simulink model "hab"  (R2024b)
settings: Solver=VariableStepAuto  StartTime=0.0  StopTime=10  RelTol=1e-3
values from neighbouring files (symbols this model uses):
  g = 9.81    [constants.m]
  h = 20000    [constants.m]
  m_balloon = 500    [constants.m]
  m_gas = 1600    [constants.m]
  M_gas = 4.002602    [constants.m]
  m_payload = 1500    [constants.m]
  R = 8.314    [constants.m]
  up = [0 0 1]    [constants.m]
libraries: shared6dof x1, aerolibatmos2 x1
settings Model: Creator=Eduard Anton  LastModifiedBy=Eduard Anton

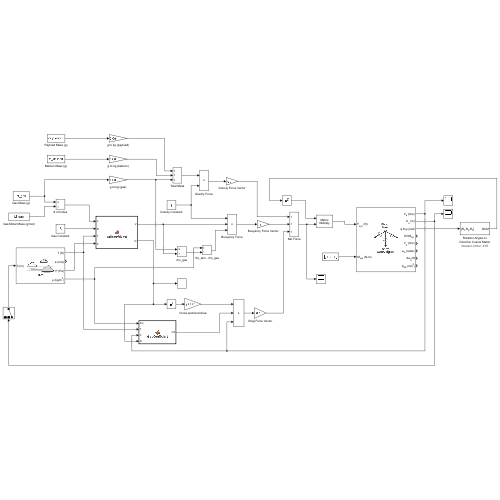
[thumbnail: Simulink's stored preview of the top-level diagram]
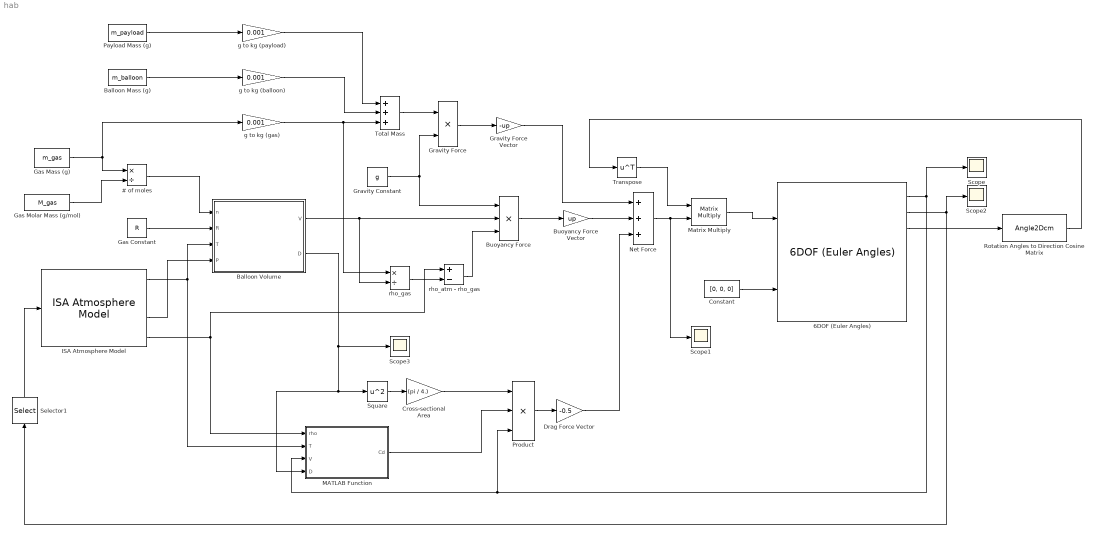
== system hab ==
  # of moles : Product  Inputs=*/
  6DOF (Euler Angles) : shared6dof/6DOF (Euler Angles)  units=Metric (MKS)  mtype=Fixed  rep=Euler Angles  xme_0=[0 0 h]  Vm_0=[0 0 0]  eul_0=[0 0 0]  pm_0=[0 0 0]  mass_0=1.0  mass_e=0.5  mass_f=2.0  inertia=eye(3)  inertia_e=eye(3)  inertia_f=2*eye(3)  k_quat=1.0  vre_flag=on  abi_flag=off  aMode=0  xme_statename=''  Vm_statename=''  eul_statename=''  quat_statename=''  pm_statename=''  mass_statename=''
  Balloon Mass (g) : Constant  Value=m_balloon
  Balloon Volume : MATLAB Function  TreatAsAtomicUnit=on
  Buoyancy Force : Product  Inputs=3
  Buoyancy Force Vector : Gain  Gain=up
  Constant : Constant  Value=[0, 0, 0]
  Cross-sectional Area : Gain  Gain=(pi / 4.)
  Drag Force Vector : Gain  Gain=-0.5
  Gas Constant : Constant  Value=R  VectorParams1D=off
  Gas Mass (g) : Constant  Value=m_gas
  Gas Molar Mass (g/mol) : Constant  Value=M_gas
  Gravity Constant : Constant  Value=g
  Gravity Force : Product
  Gravity Force Vector : Gain  Gain=-up
  ISA Atmosphere Model : aerolibatmos2/ISA Atmosphere Model  useExtended=on  action=Warning  custom=off  viscosityOut=off  g=9.80665  gamma=1.4  R=287.0531  L=0.0065  h_trop=11000  h_strat=20000  rho0=1.225  P0=101325  T0=288.15  h0=0  S=110.4  Tref=273.15  muref=1.716e-5
  MATLAB Function : MATLAB Function  TreatAsAtomicUnit=on
  Matrix Multiply : Product  Multiplication=Matrix(*)
  Net Force : Sum  Inputs=+++
  Payload Mass (g) : Constant  Value=m_payload
  Product : Product  Inputs=3
  Rotation Angles to Direction Cosine Matrix : Angle2Dcm  rotationOrder=XYZ
      settings: AttributesFormatString=Rotation Order: %<rotationOrder>
  Scope{,1..3} (4 alike) : Scope
  Selector1 : Selector  InputPortWidth=3  IndexOptions=Index vector (dialog)  Indices=3  OutputSizes=1
  Square : Math  Operator=square
  Total Mass : Sum  Inputs=+++
  Transpose : Math  Operator=transpose
  g to kg (balloon) : Gain  Gain=0.001
  g to kg (gas) : Gain  Gain=0.001
  g to kg (payload) : Gain  Gain=0.001
  rho_atm - rho_gas : Sum  Inputs=+-
  rho_gas : Product  Inputs=*/
  wires:
  ISA Atmosphere Model/1 -> Balloon Volume/3(T), MATLAB Function/2(T)
  ISA Atmosphere Model/3 -> Balloon Volume/4(P)
  Gas Constant/1 -> Balloon Volume/2(R)
  # of moles/1 -> Balloon Volume/1(n)
  ISA Atmosphere Model/4 -> rho_atm - rho_gas/1, MATLAB Function/1(rho)
  Gravity Constant/1 -> Buoyancy Force/1, Gravity Force/2
  Gas Mass (g)/1 -> g to kg (gas)/1, # of moles/1
  Gas Molar Mass (g/mol)/1 -> # of moles/2
  Balloon Volume/2(D) -> Scope3/1, MATLAB Function/4(D), Square/1
  Square/1 -> Cross-sectional Area/1
  Cross-sectional Area/1 -> Product/1
  MATLAB Function/1(Cd) -> Product/2
  Product/1 -> Drag Force Vector/1
  Constant/1 -> 6DOF (Euler Angles)/2
  g to kg (gas)/1 -> rho_gas/1, Total Mass/3
  Gravity Force/1 -> Gravity Force Vector/1
  Buoyancy Force/1 -> Buoyancy Force Vector/1
  6DOF (Euler Angles)/1 -> Product/3, MATLAB Function/3(V), Scope/1
  6DOF (Euler Angles)/2 -> Scope2/1, Selector1/1
  Balloon Volume/1(V) -> rho_gas/2, Buoyancy Force/2
  rho_gas/1 -> rho_atm - rho_gas/2
  rho_atm - rho_gas/1 -> Buoyancy Force/3
  Gravity Force Vector/1 -> Net Force/1
  Buoyancy Force Vector/1 -> Net Force/2
  Total Mass/1 -> Gravity Force/1
  Balloon Mass (g)/1 -> g to kg (balloon)/1
  g to kg (balloon)/1 -> Total Mass/2
  Payload Mass (g)/1 -> g to kg (payload)/1
  g to kg (payload)/1 -> Total Mass/1
  6DOF (Euler Angles)/3 -> Rotation Angles to Direction Cosine Matrix/1
  Net Force/1 -> Scope1/1, Matrix Multiply/2
  Rotation Angles to Direction Cosine Matrix/1 -> Transpose/1
  Transpose/1 -> Matrix Multiply/1
  Selector1/1 -> ISA Atmosphere Model/1
  Matrix Multiply/1 -> 6DOF (Euler Angles)/1
  Drag Force Vector/1 -> Net Force/3

== matlab function hab/MATLAB Function ==
  data: rho input; T input; V input; D input; Cd output
function Cd = dragCoefficient(rho, T, V, D)
    % Calculate the drag coefficient for a sphere
    % rho: air density (kg/m^3)
    % T: temperature (K)
    % V: velocity vector [x y z] (m/s)
    % D: diameter of the sphere (m)

    % If velocity is zero, set drag coefficient to zero
    V_mag = norm(V);
    if V_mag == 0
        Cd = 0;
        return;
    end

    % Compute dynamic viscosity (Sutherland's formula)
    mu = 1.716e-5 * (T / 273.15) ^ (3. / 2.) * ((273.15 + 110.4) / (T + 110.4));

    % Compute Reynolds number
    Re = (rho * V_mag * D) / mu;

    % Compute drag coefficient using formula (Morrison, 2013) Book
    term1 = 24. / Re;
    term2 = (2.6 * (Re / 5.0)) / (1 + (Re / 5.0) ^ 1.52);
    term3 = (0.411 * (Re / (2.63e5)) ^ -7.94) / (1 + (Re / (2.63e5)) ^ -8.00);
    term4 = (0.25 * (Re / 1e6)) / (1 + (Re / 1e6));
    Cd = term1 + term2 + term3 + term4;

== matlab function hab/Balloon Volume ==
  data: n input; V output; R input; T input; P input; D output
function [V, D] = balloonVolume(n, R, T, P)
    % Calculate the volume of the gas inside the balloon
    % n: amount of gas (mol)
    % R: gas constant (8.314 J/(mol·K))
    % T: temperature (K)
    % P: pressure (Pa)
    V = (n * R * T) / P;
    D = 2 * (3 * V / (4 * pi)) ^ (1. / 3.);
end
